simulink model "LQE"  (R2015a)
settings: Solver=FixedStepDiscrete  StartTime=0.0  StopTime=120  FixedStep=0.02  RelTol=1e-3
values from neighbouring files (symbols this model uses):
  A = [3.3545 -4.3521 2.6058 -0.6082; 1 0 0 0; 0 1 0 0; 0 0 1 0]    [LQGm.m]    (also in Testes_planta.m = [3.11506910744011 -3.74010634305672 2.06382118501694 -0.4387)
  B = [1;0;0;0]    [LQGm.m]    (also in Testes_planta.m)
  C = [-0.0657 0.1152 0 0]    [LQGm.m]    (also in Testes_planta.m = [-0.0767099115028891 0.161398714293952 0 0])
undefined symbols (not defined in the file or in its folder): M
settings Model: Creator=user  LastModifiedBy=user

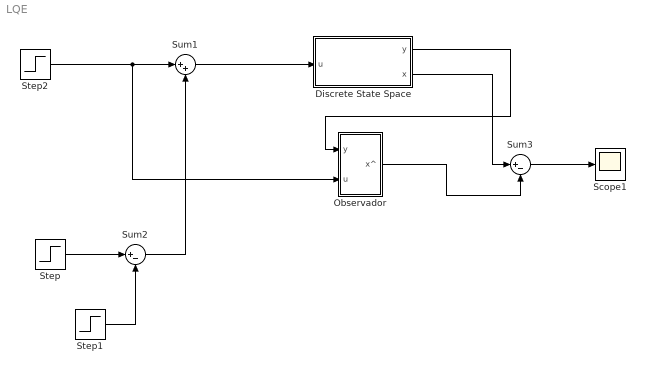
== system LQE ==
  "Discrete State Space " : Subsystem
  Observador : Subsystem
  Scope1 : Scope
  Step : Step  SampleTime=0
  Step1 : Step  Time=2  SampleTime=0
  Step2 : Step  After=0  SampleTime=0
  Sum1 : Sum  Inputs=|++
  Sum2 : Sum  Inputs=|+-
  Sum3 : Sum  Inputs=|+-
  wires:
  "Discrete State Space "/1(y) -> Observador/1(y)
  Sum1/1 -> "Discrete State Space "/1(u)
  Step2/1 -> Observador/2(u), Sum1/1
  Sum2/1 -> Sum1/2
  Step/1 -> Sum2/1
  Step1/1 -> Sum2/2
  "Discrete State Space "/2(x) -> Sum3/1
  Observador/1(x^) -> Sum3/2
  Sum3/1 -> Scope1/1

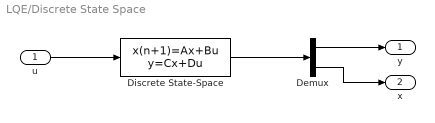
== system LQE/Discrete State Space  ==
  u : Inport
  Demux : Demux  Outputs=[1 length(A)]
  Discrete State-Space : DiscreteStateSpace  A=A  B=B  C=[C;eye(4)]  D=[0;0;0;0;0]  SampleTime=0.001
  y : Outport
  x : Outport  Port=2
  wires:
  Discrete State-Space/1 -> Demux/1
  Demux/1 -> y/1
  Demux/2 -> x/1
  u/1 -> Discrete State-Space/1

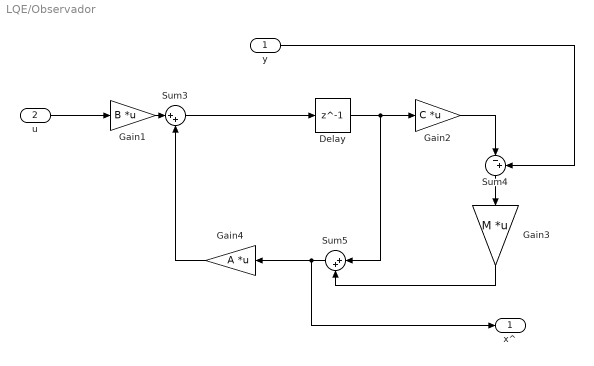
== system LQE/Observador ==
  y : Inport
  u : Inport  Port=2
  Delay : Delay  DelayLength=1  InitialCondition=0
  Gain1 : Gain  Gain=B  Multiplication=Matrix(K*u)
  Gain2 : Gain  Gain=C  Multiplication=Matrix(K*u)
  Gain3 : Gain  Gain=M  Multiplication=Matrix(K*u)
  Gain4 : Gain  Gain=A  Multiplication=Matrix(K*u)
  Sum3 : Sum  Inputs=|++
  Sum4 : Sum  Inputs=|-+
  Sum5 : Sum  Inputs=|++
  x^ : Outport
  wires:
  u/1 -> Gain1/1
  Gain1/1 -> Sum3/1
  Sum4/1 -> Gain3/1
  Gain3/1 -> Sum5/2
  Gain4/1 -> Sum3/2
  Sum5/1 -> x^/1, Gain4/1
  Delay/1 -> Sum5/1, Gain2/1
  Gain2/1 -> Sum4/1
  Sum3/1 -> Delay/1
  y/1 -> Sum4/2
